simulink model "hysteresis"  (R2021a)
settings: Solver=VariableStepAuto  StartTime=0.0  StopTime=10.0  RelTol=1e-3
libraries: eeGeneralControl x1
settings Model: Creator=lucacrupi  LastModifiedBy=lucacrupi

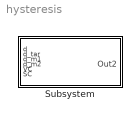
== system hysteresis ==
  Subsystem : Subsystem

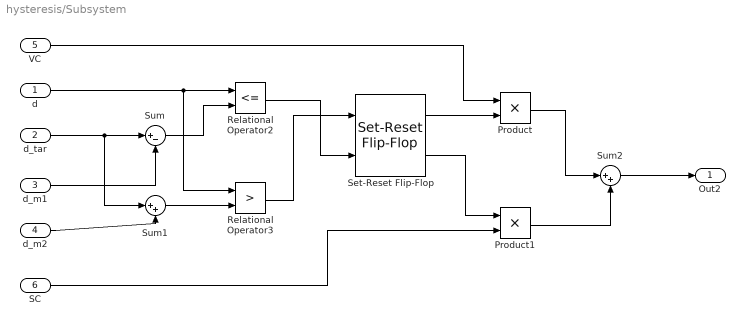
== system hysteresis/Subsystem ==
  d : Inport
  d_tar : Inport  Port=2
  d_m1 : Inport  Port=3
  d_m2 : Inport  Port=4
  VC : Inport  Port=5
  SC : Inport  Port=6
  Product : Product
  Product1 : Product
  Relational Operator2 : RelationalOperator  Operator=<=  OutDataTypeStr=boolean  RndMeth=Simplest
  Relational Operator3 : RelationalOperator  Operator=>  OutDataTypeStr=boolean  RndMeth=Simplest
  Set-Reset Flip-Flop : eeGeneralControl/Set-Reset Flip-Flop  LabelModeActiveChoice=Discrete  UndefState=Set  Q0=0  Ts=-1
      settings: SourceProductBaseCode=PS
  Sum : Sum  Inputs=|+-
  Sum1 : Sum  Inputs=|++
  Sum2 : Sum  Inputs=|++
  Out2 : Outport
  wires:
  d_m2/1 -> Sum1/2
  Sum1/1 -> Relational Operator3/2
  Relational Operator2/1 -> Set-Reset Flip-Flop/2
  VC/1 -> Product/1
  SC/1 -> Product1/2
  Relational Operator3/1 -> Set-Reset Flip-Flop/1
  Sum/1 -> Relational Operator2/2
  d_m1/1 -> Sum/2
  d/1 -> Relational Operator3/1, Relational Operator2/1
  d_tar/1 -> Sum1/1, Sum/1
  Product1/1 -> Sum2/2
  Product/1 -> Sum2/1
  Sum2/1 -> Out2/1
  Set-Reset Flip-Flop/1 -> Product/2
  Set-Reset Flip-Flop/2 -> Product1/1
